simulink model "s360159_sim"  (R2025b)
settings: Solver=VariableStepAuto  StartTime=0.0  StopTime=t_sim  RelTol=1e-3
values from neighbouring files (symbols this model uses):
  d1 = 0    [s360159.mat]    (also in s360159_design.m)
  d2 = 0    [s360159.mat]    (also in s360159_design.m)
  r = 1    [s360159.mat]    (also in s360159_design.m)
  Ts = 0.005    [s360159.mat]    (also in s360159_MPC.mat = 0.05; s360159_design.m)
libraries: cstblocks x2
settings Model: Creator=giovannimasi  LastModifiedBy=giovannimasi

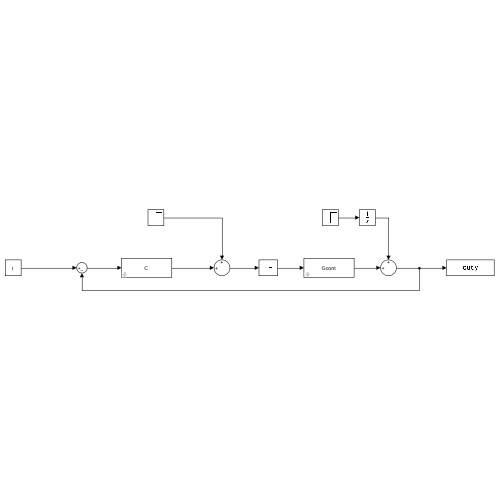
[thumbnail: Simulink's stored preview of the top-level diagram]
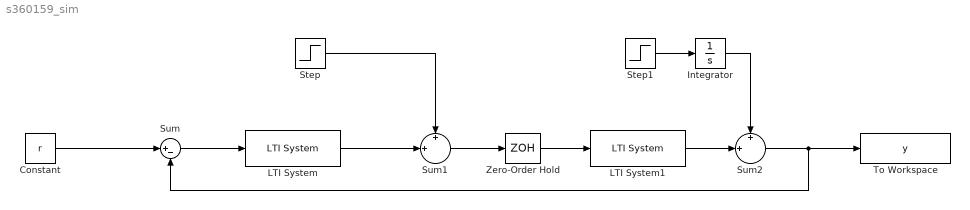
== system s360159_sim ==
  Constant : Constant  Value=r  SampleTime=Ts
  Integrator : Integrator
  LTI System : cstblocks/LTI System  sys=C  IC=[]  PadeOrder=0
  LTI System1 : cstblocks/LTI System  sys=Gcont  IC=[]  PadeOrder=0
  Step : Step  Time=0  After=d1  SampleTime=Ts
  Step1 : Step  Time=0  After=d2  SampleTime=Ts
  Sum : Sum  Inputs=|+-
  Sum1 : Sum  Inputs=+|+||
  Sum2 : Sum  Inputs=+|+||
  To Workspace : ToWorkspace  VariableName=y  SaveFormat=Timeseries  SampleTime=Ts
  Zero-Order Hold : ZeroOrderHold  SampleTime=Ts
  wires:
  Constant/1 -> Sum/1
  Sum/1 -> LTI System/1
  LTI System/1 -> Sum1/2
  Step/1 -> Sum1/1
  Sum1/1 -> Zero-Order Hold/1
  Zero-Order Hold/1 -> LTI System1/1
  LTI System1/1 -> Sum2/2
  Step1/1 -> Integrator/1
  Integrator/1 -> Sum2/1
  Sum2/1 -> Sum/2, To Workspace/1
